simulink model "manyUnitDelay"  (R2014a)
settings: Solver=FixedStepDiscrete  StartTime=0.0  StopTime=10.0  FixedStep=0.1  RelTol=1e-3
settings Model: Creator=yoshi12  LastModifiedBy=yoshi12

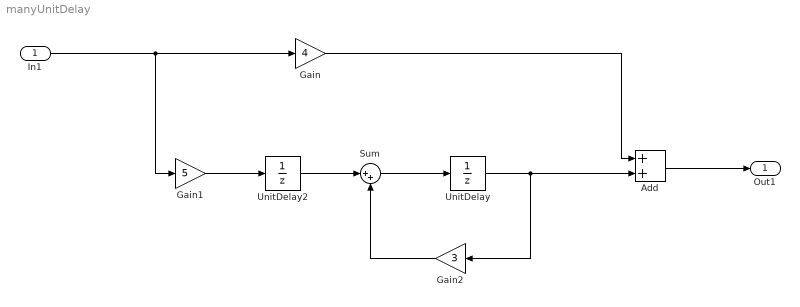
== system manyUnitDelay ==
  In1 : Inport
  Add : Sum
  Gain : Gain  Gain=4
  Gain1 : Gain  Gain=5
  Gain2 : Gain  Gain=3
  Sum : Sum  Inputs=|++
  UnitDelay : UnitDelay  SampleTime=-1
  UnitDelay2 : UnitDelay  SampleTime=-1
  Out1 : Outport
  wires:
  In1/1 -> Gain1/1, Gain/1
  Gain/1 -> Add/1
  Add/1 -> Out1/1
  Gain1/1 -> UnitDelay2/1
  UnitDelay/1 -> Add/2, Gain2/1
  Gain2/1 -> Sum/2
  UnitDelay2/1 -> Sum/1
  Sum/1 -> UnitDelay/1
